simulink model "PSKyangyufei6_5"  (Simulink 5.0)
settings: Solver=ode45  StartTime=0.0  StopTime=10.0  RelTol=1e-3
libraries: commchan2 x1, dsparch4 x1, commrandsrc2 x1, commsink2 x1, dspsigops x1
settings Model: LastModifiedBy=lenovo

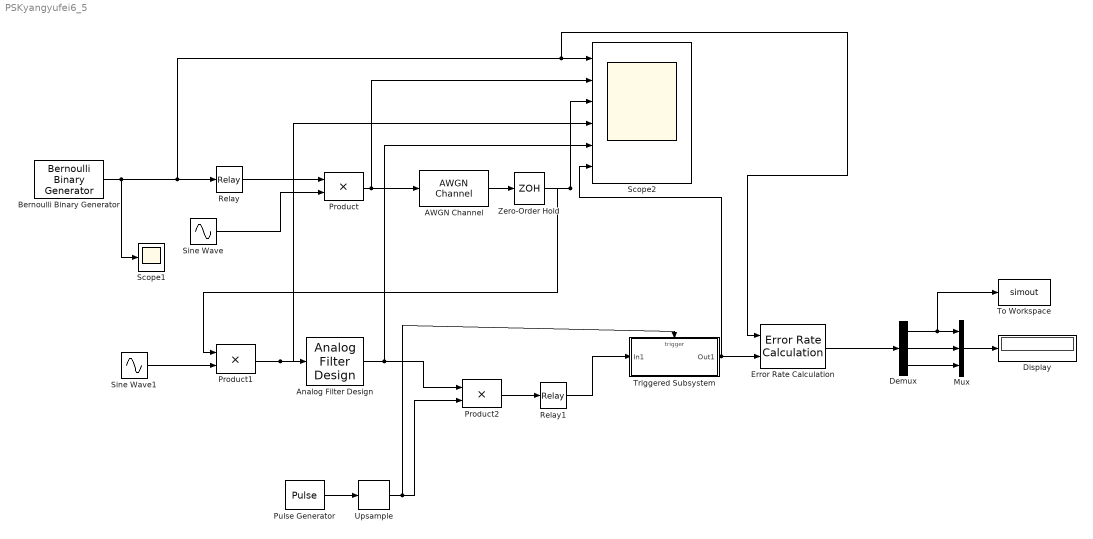
== system PSKyangyufei6_5 ==
  AWGN Channel : commchan2/AWGN Channel  seed=67  noiseMode="Signal to noise ratio  (SNR)"  EsNodB=10  SNRdB=10  Ps=1  Tsym=1  variance=1
  Analog Filter Design : dsparch4/Analog Filter Design  method=Butterworth  filttype=Lowpass  N=2  Wlo=2*pi*2  Whi=80  Rp=2  Rs=40
  Bernoulli Binary Generator : commrandsrc2/Bernoulli Binary Generator  P=0.5  seed=61  Ts=0.5  frameBased=off  sampPerFrame=1  orient=off
  Demux : Demux  Outputs=3
  Display : Display
  Error Rate Calculation : commsink2/Error Rate Calculation  N=0  st_delay=0  cp_mode=Entire frame  subframe=[]  PMode=Port  WsName=ErrorVec  RsMode2=off  stop=off  numErr=100  maxBits=1e6
  Mux : Mux  Inputs=3
  Product : Product  SaturateOnIntegerOverflow=on
  Product1 : Product  SaturateOnIntegerOverflow=on
  Product2 : Product  SaturateOnIntegerOverflow=on
  Pulse Generator : DiscretePulseGenerator  Period=10  PulseWidth=5  SampleTime=1/500
  Relay : Relay  OnSwitchValue=0.1  OffSwitchValue=0.1  OffOutputValue=-1
  Relay1 : Relay  OnSwitchValue=0.1  OffSwitchValue=0.1
  Scope1 : Scope
  Scope2 : Scope  NumInputPorts=6
      settings: YMin=0~-5~-5~-5~-5~0  YMax=1~5~5~5~5~1
  Sine Wave : Sin  Amplitude=2  Frequency=2*pi*10  Samples=2*pi*20  SampleTime=1/500
  Sine Wave1 : Sin  Amplitude=2  Frequency=2*pi*10  SampleTime=1/500
  To Workspace : ToWorkspace  VariableName=simout  SampleTime=-1  SaveFormat=Structure
  Triggered Subsystem : Subsystem  TreatAsAtomicUnit=on
  Upsample : dspsigops/Upsample  N=10  phase=0  ic=0  mode=Maintain input frame size
  Zero-Order Hold : ZeroOrderHold  SampleTime=1/500
  wires:
  Bernoulli Binary Generator/1 -> Error Rate Calculation/1, Scope2/1, Relay/1, Scope1/1
  Relay/1 -> Product/1
  Sine Wave/1 -> Product/2
  Product/1 -> AWGN Channel/1, Scope2/2
  Sine Wave1/1 -> Product1/2
  Product2/1 -> Relay1/1
  Relay1/1 -> Triggered Subsystem/1(In1)
  Pulse Generator/1 -> Upsample/1
  Upsample/1 -> Triggered Subsystem/Trigger, Product2/2
  Triggered Subsystem/1(Out1) -> Error Rate Calculation/2, Scope2/6
  Error Rate Calculation/1 -> Demux/1
  Demux/1 -> Mux/1, To Workspace/1
  Demux/2 -> Mux/2
  Demux/3 -> Mux/3
  Mux/1 -> Display/1
  Product1/1 -> Analog Filter Design/1, Scope2/4
  Analog Filter Design/1 -> Product2/1, Scope2/5
  Zero-Order Hold/1 -> Product1/1, Scope2/3
  AWGN Channel/1 -> Zero-Order Hold/1

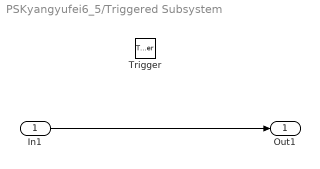
== system PSKyangyufei6_5/Triggered Subsystem ==
  In1 : Inport
  Trigger : TriggerPort
  Out1 : Outport
  wires:
  In1/1 -> Out1/1
